simulink model "limited_time_undereacted_spacecraft_change"  (R2022a)
settings: Solver=ode4  StartTime=0.0  StopTime=30  FixedStep=0.001  RelTol=1e-11
libraries: simulink x4
settings Model: Creator=田佳怡  LastModifiedBy=lyuwenhao
settings SolverCC: AlgebraicLoopSolver=TrustRegion
settings DebuggingCC: UnconnectedInputMsg=warning  UnconnectedOutputMsg=warning  UnconnectedLineMsg=warning  SFMachineParentedDataDiag=warning
settings RTWCC: DLArmComputeVersion=19.05

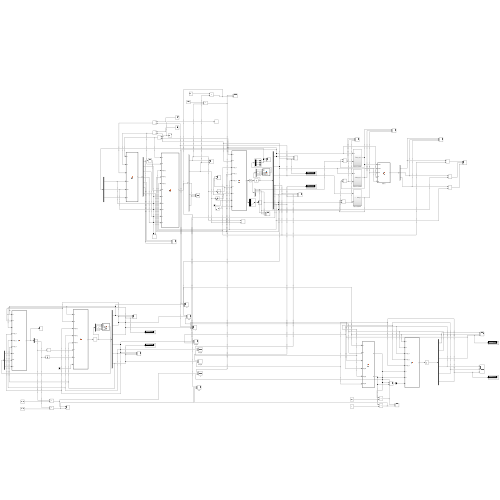
[thumbnail: Simulink's stored preview of the top-level diagram]
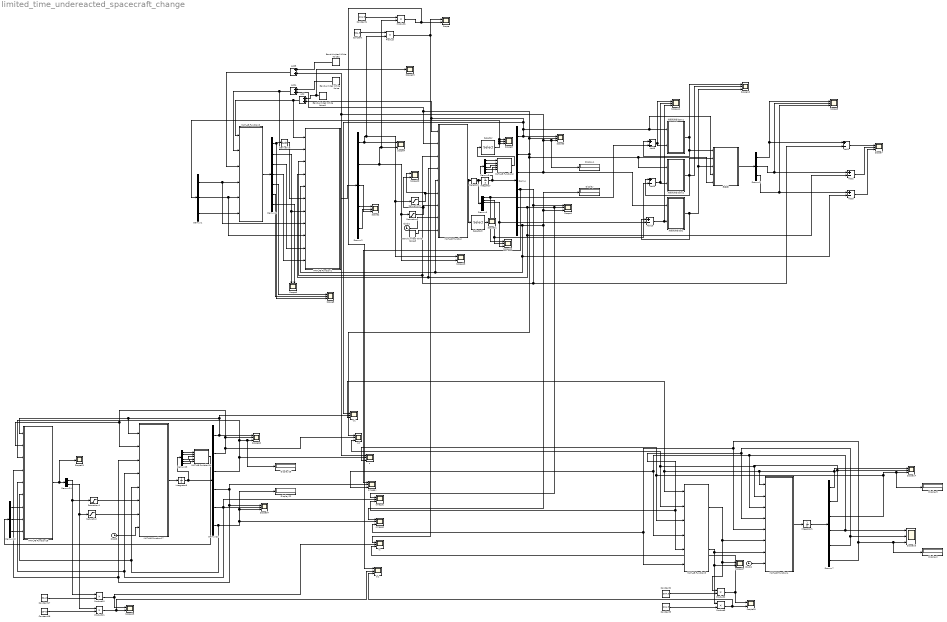
== system limited_time_undereacted_spacecraft_change ==
  Add : Sum
  Add{1..3,8..10} (6 alike) : Sum  Inputs=+-
  Add4 : Sum
  Add5 : Sum
  Band-Limited White Noise : simulink/Sources/Band-Limited White Noise  Cov=[0.001*0.001*0.0001]  Ts=0.01  seed=[23341]
  Band-Limited White Noise1 : simulink/Sources/Band-Limited White Noise  Cov=[0.001*0.001*0.0001]  Ts=0.01  seed=[23341]
  Band-Limited White Noise2 : simulink/Sources/Band-Limited White Noise  Cov=[0.001*0.001*0.0001]  Ts=0.1  seed=[23341]
  Band-Limited White Noise3 : simulink/Sources/Band-Limited White Noise  Cov=[0.001*0.001*0.0001]  Ts=0.01  seed=[23341]
  Clock1 : Clock
  Clock2 : Clock
  Clock3 : Clock
  Constant : Constant  Value=304.5
  Constant1 : Constant  Value=204.5
  Constant17 : Constant  Value=304.5
  Constant18 : Constant  Value=204.5
  Constant2 : Constant  Value=304.5
  Constant3 : Constant  Value=204.5
  Demux{,3,6..7,21,23} (6 alike) : Demux  Outputs=6
  Demux1 : Demux  Outputs=3
  Demux2 : Demux  Outputs=5
  Demux22 : Demux  Outputs=3
  Demux24 : Demux  Outputs=2
  Demux4 : Demux  Outputs=7
  Demux5 : Demux  Outputs=3
  Derivative : Derivative
  Display{,1..2,5,22,25} (6 alike) : Display
  Integrator : Integrator  InitialCondition=[2.5;2.5;-0.213175;0.1;-0.1;-0.15095622]
  Integrator1 : Integrator  InitialCondition=[2;2;0.428875;0.2;-0.2;-0.12250622]
  Integrator9 : Integrator  InitialCondition=[2;2;0.428875;0.2;-0.2;-0.12250622]
  MATLAB Function : MATLAB Function  TreatAsAtomicUnit=on
  MATLAB Function1 : MATLAB Function  TreatAsAtomicUnit=on
  MATLAB Function17 : MATLAB Function  TreatAsAtomicUnit=on
  MATLAB Function18 : MATLAB Function  TreatAsAtomicUnit=on
  MATLAB Function19 : MATLAB Function  TreatAsAtomicUnit=on
  MATLAB Function2 : MATLAB Function  TreatAsAtomicUnit=on
  MATLAB Function3 : MATLAB Function  TreatAsAtomicUnit=on
  MATLAB Function4 : MATLAB Function  TreatAsAtomicUnit=on
  MATLAB Function5 : MATLAB Function  TreatAsAtomicUnit=on
  Product{,1..3,10..11} (6 alike) : Product
  Saturation{,1..3} (4 alike) : Saturate
  Scope{,4,6,13,15,17..18,20} (8 alike) : Scope  NumInputPorts=2
  Scope{1..3,5,7..12,14,16,57,60} (14 alike) : Scope  NumInputPorts=3
  Scope19 : Scope
  Scope21 : Scope
  Scope61 : Scope
  Selector : Selector  InputPortWidth=3  IndexOptions=Index vector (dialog)  Indices=[1 2 3]  OutputSizes=1
  Selector1 : Selector  InputPortWidth=7  IndexOptions=Index vector (dialog)  Indices=[1 2 3 4 5 6]  OutputSizes=1
  Selector2 : Selector  InputPortWidth=7  IndexOptions=Index vector (dialog)  Indices=[7]  OutputSizes=1
  omegax : Scope  NumInputPorts=3
  omegay : Scope  NumInputPorts=3
  omegaz : Scope  NumInputPorts=3
  tx : Scope  NumInputPorts=3
  tx1 : Scope  NumInputPorts=3
  w1 : Scope  NumInputPorts=3
  w2 : Scope  NumInputPorts=3
  z : Scope  NumInputPorts=3
  滑膜观测器dotw1 : Subsystem
  滑膜观测器dotw2 : Subsystem
  滑膜观测器dotz : Subsystem
  角速度 : MATLAB Function  TreatAsAtomicUnit=on
  wires:
  Demux/3 -> z/1, Add5/2, Display1/1, Scope3/3, 滑膜观测器dotz/1(z)
  Demux/2 -> w2/1, 滑膜观测器dotw2/1(w2), 角速度/5(w2), Scope3/2, MATLAB Function/2(w2), Add4/2
  MATLAB Function1/1(y) -> Demux2/1
  MATLAB Function2/1(y) -> Selector/1
  Demux3/1 -> MATLAB Function2/1(w1)
  Demux3/2 -> MATLAB Function2/2(w2)
  Demux3/4 -> MATLAB Function2/3(omega_x)
  Demux3/5 -> MATLAB Function2/4(omega_y)
  Demux3/6 -> MATLAB Function2/5(omega_z)
  MATLAB Function3/1(y) -> Demux4/1
  Demux1/2 -> MATLAB Function1/9(dw2), MATLAB Function3/5(dw2)
  Demux1/1 -> MATLAB Function1/8(dw1), MATLAB Function3/4(dw1)
  Demux1/3 -> MATLAB Function3/6(dz)
  Demux4/1 -> Derivative/1, Scope5/3
  Derivative/1 -> MATLAB Function1/6(dz3)
  Demux4/2 -> MATLAB Function1/7(s2), Scope6/1
  Demux/4 -> Add1/2, MATLAB Function/3(omega_x), MATLAB Function1/3(omega_x), Scope1/1, omegax/1
  Demux4/3 -> MATLAB Function1/10(h1)
  Demux4/4 -> MATLAB Function1/11(h2)
  Constant/1 -> Product/1
  Product/1 -> Scope/1, tx/1
  Constant1/1 -> Product1/1
  Demux2/5 -> Scope2/2
  Demux2/4 -> Scope2/1
  Demux2/3 -> Scope2/3
  Demux4/5 -> Scope5/1
  Demux4/6 -> Scope5/2
  Selector/1 -> Scope8/3, Scope8/2, Scope8/1, Demux1/1
  Integrator/1 -> Demux/1, Demux3/1
  Demux5/3 -> Scope9/3, Add3/1
  角速度/1(y) -> Demux5/1
  Demux5/2 -> Scope9/2, Add2/1
  Demux5/1 -> Scope9/1, Add1/1
  Add8/1 -> Scope11/1, 滑膜观测器dotw1/2(In1)
  MATLAB Function/1(y) -> Selector2/1, Selector1/1
  Demux6/1 -> Scope12/1, Add8/2
  滑膜观测器dotw1/1(dotw_1估计) -> Scope10/1, 角速度/1(dotw1), Add8/1
  Add9/1 -> Scope11/2, 滑膜观测器dotw2/2(In1)
  Demux6/2 -> Scope12/2, Add9/2
  Add10/1 -> Scope11/3, 滑膜观测器dotz/2(In1)
  滑膜观测器dotz/1(dotz估计) -> Scope10/3, 角速度/3(dotz), Add10/1
  Demux6/3 -> Scope12/3, Add10/2
  滑膜观测器dotw2/1(dotw_2估计) -> 角速度/2(dotw2), Scope10/2, Add9/1
  Demux/6 -> Add3/2, MATLAB Function/5(omega_z), MATLAB Function1/5(omega_z), Display/1, Scope1/3, omegaz/1
  Add1/1 -> Scope7/1
  Add2/1 -> Scope7/2
  Add3/1 -> Scope7/3
  Demux4/7 -> Scope6/2
  Product11/1 -> tx1/2, Scope15/2
  Demux23/1 -> MATLAB Function19/1(w1)
  Demux22/3 -> MATLAB Function18/9(dz)
  Integrator9/1 -> Demux23/1, Demux21/1
  Demux22/1 -> MATLAB Function18/7(dw1)
  Demux21/4 -> MATLAB Function18/4(omega_x), MATLAB Function17/3(omega_x), Scope57/1, omegax/2
  Demux21/3 -> z/2, MATLAB Function18/3(z), Display25/1, Scope60/3
  MATLAB Function18/1(y) -> Scope61/1, Demux24/1
  Demux23/2 -> MATLAB Function19/2(w2)
  Constant17/1 -> Product10/2
  MATLAB Function17/1(y) -> Integrator9/1
  Demux22/2 -> MATLAB Function18/8(dw2)
  Demux23/4 -> MATLAB Function19/3(omega_x)
  MATLAB Function19/1(y) -> Demux22/1
  Demux24/1 -> Product10/1, Saturation1/1
  Demux24/2 -> Product11/1, Saturation/1
  Demux21/6 -> MATLAB Function17/5(omega_z), MATLAB Function18/6(omega_z), Display22/1, Scope57/3, omegaz/2
  Demux21/1 -> Scope60/1, w1/2, MATLAB Function18/1(w1), MATLAB Function17/1(w1)  "w1"
  Demux21/2 -> w2/2, Scope60/2, MATLAB Function18/2(w2), MATLAB Function17/2(w2)  "w2"
  Demux21/5 -> MATLAB Function17/4(omega_y), MATLAB Function18/5(omega_y), omegay/2, Scope57/2
  Constant18/1 -> Product11/2
  Demux23/6 -> MATLAB Function19/5(omega_z)
  Demux23/5 -> MATLAB Function19/4(omega_y)
  Demux7/2 -> MATLAB Function5/2(w2), w2/3, MATLAB Function4/2(w2), Scope14/2
  Demux7/1 -> MATLAB Function5/1(w1), w1/3, MATLAB Function4/1(w1), Scope14/1
  Demux7/3 -> MATLAB Function5/3(z), z/3, Display5/1, Scope14/3
  Clock2/1 -> MATLAB Function4/8(t)
  Demux7/6 -> MATLAB Function4/5(omega_z), MATLAB Function5/6(omegaz), omegaz/3, Display2/1, Scope16/3
  Integrator1/1 -> Demux7/1
  MATLAB Function4/1(y) -> Integrator1/1
  Demux/1 -> w1/1, MATLAB Function/1(w1), Add/2, 角速度/4(w1), 滑膜观测器dotw1/1(w1), Scope3/1
  Demux7/4 -> MATLAB Function4/3(omega_x), MATLAB Function5/4(omegax), omegax/3, Scope16/1
  Demux/5 -> Add2/2, MATLAB Function/4(omega_y), MATLAB Function1/4(omega_y), omegay/1, Scope1/2
  Demux7/5 -> MATLAB Function5/5(omegay), omegay/3, MATLAB Function4/4(omega_y), Scope16/2
  Product10/1 -> Scope15/1, tx/2
  Product2/1 -> Scope18/1, tx/3
  Constant3/1 -> Product3/2
  MATLAB Function5/2(u2) -> MATLAB Function4/7(u2), Product3/1, Scope17/2
  Constant2/1 -> Product2/2
  MATLAB Function5/1(u1) -> MATLAB Function4/6(u1), Product2/1, Scope17/1
  Product3/1 -> tx1/3, Scope18/2
  Product1/1 -> tx1/1, Scope/2
  Demux2/1 -> Scope13/1, Saturation3/1, Product/2, Scope4/1
  Demux2/2 -> Scope13/2, Saturation2/1, Scope4/2, Product1/2
  Clock1/1 -> MATLAB Function/8(t)
  Clock3/1 -> MATLAB Function17/8(t)
  Saturation1/1 -> MATLAB Function17/6(u1)
  Saturation/1 -> MATLAB Function17/7(u2)
  Band-Limited White Noise/1 -> Add4/1
  Band-Limited White Noise1/1 -> Scope19/1, Add/1
  Add/1 -> MATLAB Function3/1(w1), MATLAB Function1/1(w1)
  Add4/1 -> MATLAB Function3/2(w2), MATLAB Function1/2(w2)
  Band-Limited White Noise2/1 -> Add5/1
  Add5/1 -> MATLAB Function3/3(z)
  Saturation2/1 -> Scope20/2, MATLAB Function/7(u2)
  Saturation3/1 -> MATLAB Function/6(u1), Scope20/1
  Selector1/1 -> Demux6/1, Integrator/1
  Selector2/1 -> Scope21/1
  Band-Limited White Noise3/1 -> MATLAB Function/9(d)

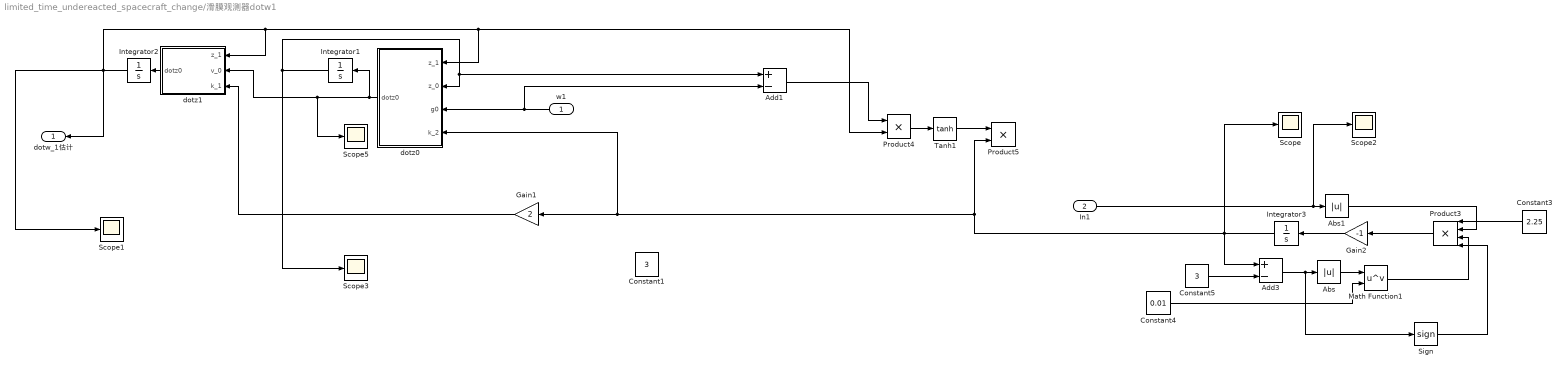
== system limited_time_undereacted_spacecraft_change/滑膜观测器dotw1 ==
  w1 : Inport
  In1 : Inport  Port=2
  Abs : Abs  SaturateOnIntegerOverflow=off
  Abs1 : Abs  SaturateOnIntegerOverflow=off
  Add1 : Sum  Inputs=+-
  Add3 : Sum  Inputs=+-
  Constant1 : Constant  Value=3
  Constant3 : Constant  Value=2.25
  Constant4 : Constant  Value=0.01
  Constant5 : Constant  Value=3
  Gain1 : Gain  Gain=2
  Gain2 : Gain  Gain=-1
  Integrator1 : Integrator
  Integrator2 : Integrator
  Integrator3 : Integrator  InitialCondition=8
  Math Function1 : Math  Operator=pow
  Product3 : Product  Inputs=4
  Product4 : Product
  Product5 : Product
  Scope{,1..3,5} (5 alike) : Scope
  Sign : Signum
  Tanh1 : Trigonometry  Operator=tanh
  dotz0 : MATLAB Function  TreatAsAtomicUnit=on
  dotz1 : MATLAB Function  TreatAsAtomicUnit=on
  dotw_1估计 : Outport
  wires:
  Tanh1/1 -> Product5/1
  Constant5/1 -> Add3/2
  Constant4/1 -> Math Function1/2
  w1/1 -> Add1/2, dotz0/3(g0)
  Product3/1 -> Gain2/1
  Constant3/1 -> Product3/1
  Gain2/1 -> Integrator3/1
  Add3/1 -> Sign/1, Abs/1
  Add1/1 -> Product4/1
  Integrator1/1 -> Scope3/1, dotz0/2(z_0), Add1/1
  Gain1/1 -> dotz1/3(k_1)
  Integrator2/1 -> dotw_1估计/1, Scope1/1, dotz0/1(z_1), Product4/2, dotz1/1(z_1)
  dotz1/1(dotz0) -> Integrator2/1
  In1/1 -> Scope2/1, Abs1/1
  Product4/1 -> Tanh1/1
  dotz0/1(dotz0) -> dotz1/2(v_0), Scope5/1, Integrator1/1
  Abs1/1 -> Product3/2
  Math Function1/1 -> Product3/3
  Abs/1 -> Math Function1/1
  Sign/1 -> Product3/4
  Integrator3/1 -> Scope/1, dotz0/4(k_2), Gain1/1, Product5/2, Add3/1

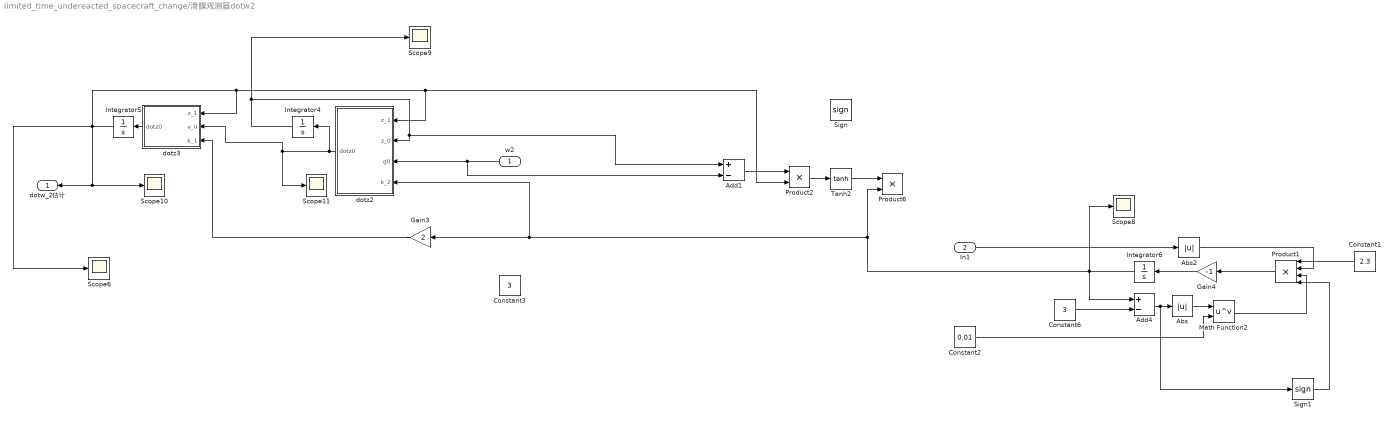
== system limited_time_undereacted_spacecraft_change/滑膜观测器dotw2 ==
  w2 : Inport
  In1 : Inport  Port=2
  Abs : Abs  SaturateOnIntegerOverflow=off
  Abs2 : Abs  SaturateOnIntegerOverflow=off
  Add1 : Sum  Inputs=+-
  Add4 : Sum  Inputs=+-
  Constant1 : Constant  Value=2.3
  Constant2 : Constant  Value=0.01
  Constant3 : Constant  Value=3
  Constant6 : Constant  Value=3
  Gain3 : Gain  Gain=2
  Gain4 : Gain  Gain=-1
  Integrator4 : Integrator
  Integrator5 : Integrator
  Integrator6 : Integrator  InitialCondition=8
  Math Function2 : Math  Operator=pow
  Product1 : Product  Inputs=4
  Product2 : Product
  Product6 : Product
  Scope{6,8..11} (5 alike) : Scope
  Sign : Signum
  Sign1 : Signum
  Tanh2 : Trigonometry  Operator=tanh
  dotz2 : MATLAB Function  TreatAsAtomicUnit=on
  dotz3 : MATLAB Function  TreatAsAtomicUnit=on
  dotw_2估计 : Outport
  wires:
  Tanh2/1 -> Product6/1
  Constant6/1 -> Add4/2
  Constant2/1 -> Math Function2/2
  w2/1 -> Add1/2, dotz2/3(g0)
  Product1/1 -> Gain4/1
  Constant1/1 -> Product1/1
  Gain4/1 -> Integrator6/1
  Add4/1 -> Sign1/1, Abs/1
  Add1/1 -> Product2/1
  Integrator4/1 -> Scope9/1, Add1/1, dotz2/2(z_0)
  Gain3/1 -> dotz3/3(k_1)
  Integrator5/1 -> dotw_2估计/1, Scope10/1, Scope6/1, dotz2/1(z_1), Product2/2, dotz3/1(z_1)
  dotz3/1(dotz0) -> Integrator5/1
  In1/1 -> Abs2/1
  Math Function2/1 -> Product1/3
  Product2/1 -> Tanh2/1
  Integrator6/1 -> dotz2/4(k_2), Gain3/1, Product6/2, Add4/1, Scope8/1
  dotz2/1(dotz0) -> dotz3/2(v_0), Scope11/1, Integrator4/1
  Abs2/1 -> Product1/2
  Abs/1 -> Math Function2/1
  Sign1/1 -> Product1/4

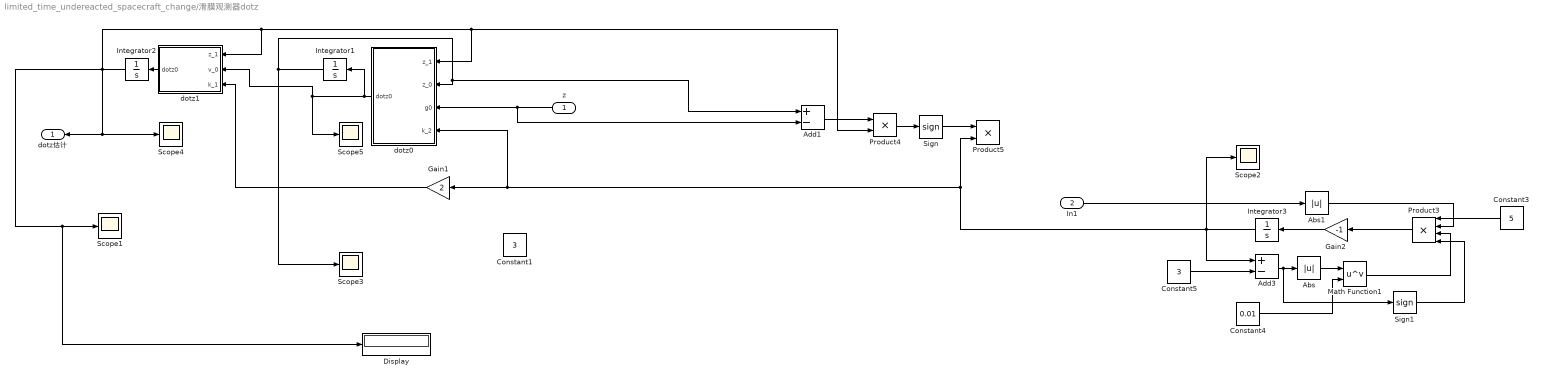
== system limited_time_undereacted_spacecraft_change/滑膜观测器dotz ==
  z : Inport
  In1 : Inport  Port=2
  Abs : Abs  SaturateOnIntegerOverflow=off
  Abs1 : Abs  SaturateOnIntegerOverflow=off
  Add1 : Sum  Inputs=+-
  Add3 : Sum  Inputs=+-
  Constant1 : Constant  Value=3
  Constant3 : Constant  Value=5
  Constant4 : Constant  Value=0.01
  Constant5 : Constant  Value=3
  Display : Display
  Gain1 : Gain  Gain=2
  Gain2 : Gain  Gain=-1
  Integrator1 : Integrator
  Integrator2 : Integrator
  Integrator3 : Integrator  InitialCondition=8
  Math Function1 : Math  Operator=pow
  Product3 : Product  Inputs=4
  Product4 : Product
  Product5 : Product
  Scope{1..5} (5 alike) : Scope
  Sign : Signum
  Sign1 : Signum
  dotz0 : MATLAB Function  TreatAsAtomicUnit=on
  dotz1 : MATLAB Function  TreatAsAtomicUnit=on
  dotz估计 : Outport
  wires:
  dotz0/1(dotz0) -> dotz1/2(v_0), Scope5/1, Integrator1/1
  dotz1/1(dotz0) -> Integrator2/1
  Gain1/1 -> dotz1/3(k_1)
  Product4/1 -> Sign/1
  Integrator1/1 -> Scope3/1, Add1/1, dotz0/2(z_0)
  z/1 -> Add1/2, dotz0/3(g0)
  Sign/1 -> Product5/1
  Add1/1 -> Product4/1
  Integrator2/1 -> dotz估计/1, Scope4/1, Display/1, Scope1/1, dotz0/1(z_1), Product4/2, dotz1/1(z_1)
  Integrator3/1 -> dotz0/4(k_2), Gain1/1, Product5/2, Add3/1, Scope2/1
  Constant4/1 -> Math Function1/2
  Math Function1/1 -> Product3/3
  Add3/1 -> Sign1/1, Abs/1
  In1/1 -> Abs1/1
  Abs1/1 -> Product3/2
  Constant5/1 -> Add3/2
  Gain2/1 -> Integrator3/1
  Constant3/1 -> Product3/1
  Product3/1 -> Gain2/1
  Abs/1 -> Math Function1/1
  Sign1/1 -> Product3/4

== matlab function limited_time_undereacted_spacecraft_change/MATLAB Function5 ==
  data: w1 input; u1 output; w2 input; z input; omegax input; omegay input; omegaz input; u2 output
function [u1, u2] = fcn(w1, w2, z, omegax, omegay, omegaz)

J3 = 403.6; J1= 304.5; J2 = 204.5; a1 = (J2 - J3) / J1; a2 = (J3 - J1) / J2; a3 = (J1 - J2) / J3;
k1 = 0.5; k2 = 0.5; k3 = 2; m = 10; n = 5; ks = 0.8; epsilon = 0.01;

v1 = omegax+k1*w1;
v2 = omegay+k2*w2;

u_eq1 = -k1*(w2*omegaz + 0.5*(1+w1^2-w2^2)*omegax + w1*w2*omegay) - ks*v1-epsilon*tanh(v1) - a1*omegay*omegaz;

u_eq2 = -k2*(-w1*omegaz + 0.5*(1-w1^2+w2^2)*omegay + w1*w2*omegax) - ks*v2-epsilon*tanh(v2) - a2*omegax*omegaz;

% us = (-ks*s2-epsilon*sign(s2)-h2*v3_dot) / (R_omegax+h1*R_omegay);

u1 = u_eq1;
u2 = u_eq2;

end

== matlab function limited_time_undereacted_spacecraft_change/滑膜观测器dotw1/dotz0 ==
  data: z_1 input; z_0 input; dotz0 output; g0 input; k_2 input
function dotz0 = fcn(z_1, z_0, g0, k_2)

v_0 = z_1 - k_2*abs(z_0 - g0)^(0.5)*tanh(z_0 - g0);


dotz0 = v_0;

== matlab function limited_time_undereacted_spacecraft_change/滑膜观测器dotw1/dotz1 ==
  data: z_1 input; dotz0 output; v_0 input; k_1 input
function dotz0 = fcn(z_1, v_0, k_1)


u = -k_1*tanh(z_1 - v_0);


dotz0 = u;

== matlab function limited_time_undereacted_spacecraft_change/滑膜观测器dotw2/dotz2 ==
  data: z_1 input; z_0 input; dotz0 output; g0 input; k_2 input
function dotz0 = fcn(z_1, z_0, g0, k_2)

v_0 = z_1 - k_2*abs(z_0 - g0)^(0.5)*tanh(z_0 - g0);


dotz0 = v_0;

== matlab function limited_time_undereacted_spacecraft_change/滑膜观测器dotw2/dotz3 ==
  data: z_1 input; dotz0 output; v_0 input; k_1 input
function dotz0 = fcn(z_1, v_0, k_1)


u = -k_1*tanh(z_1 - v_0);


dotz0 = u;

== matlab function limited_time_undereacted_spacecraft_change/滑膜观测器dotz/dotz0 ==
  data: z_1 input; z_0 input; dotz0 output; g0 input; k_2 input
function dotz0 = fcn(z_1, z_0, g0, k_2)

v_0 = z_1 - k_2*abs(z_0 - g0)^(0.5)*tanh(z_0 - g0);


dotz0 = v_0;

== matlab function limited_time_undereacted_spacecraft_change/滑膜观测器dotz/dotz1 ==
  data: z_1 input; dotz0 output; v_0 input; k_1 input
function dotz0 = fcn(z_1, v_0, k_1)


u = -k_1*tanh(z_1 - v_0);


dotz0 = u;

== matlab function limited_time_undereacted_spacecraft_change/角速度 ==
  data: dotw1 input; y output; dotw2 input; dotz input; w1 input; w2 input
function y = fcn(dotw1, dotw2, dotz, w1, w2)

% if(data<0.155)
    omega1 = (2*dotw1 - 2*dotz*w2 ) / (1+w1^2+w2^2);

    omega2 = (2*dotw2 + 2*dotz*w1 ) / (1+w1^2+w2^2);

    omega3 = dotz-w1*omega2+w2*omega1;
% else
%      omega1 = (2*dotw1-w2*(2*dotz-4*w1*dotw2)+4*w1^2*dotw1)/(1+w1^2+w2^2) - (4*w1*(w1*dotw1+w2*dotw2))/(w1^2+w2^2);
% 
%      omega2 = (2*dotw2-w1*(2*dotz+4*dotw1*w2)+4*w2^2*dotw2)/(1+w1^2+w2^2) - (4*w2*(w1*dotw1+w2*dotw2))/(w1^2+w2^2);
% 
%      omega3 = dotz-2*(dotz*w1^2+dotw2*w1+dotz*w2^2-dotw1*w2);
% end
    

y = [omega1; omega2; omega3];

== matlab function limited_time_undereacted_spacecraft_change/MATLAB Function17 ==
  data: w1 input; y output; w2 input; omega_x input; omega_y input; omega_z input; u1 input; u2 input; t input
function y = fcn(w1,w2,omega_x,omega_y,omega_z,u1,u2, t)

Jx = 304.5; Jy = 403.6; Jz = 204.5;

w1_dot = w2*omega_z + 0.5*(1+w1^2-w2^2)*omega_x + w1*w2*omega_y;
w2_dot = -w1*omega_z + 0.5*(1-w1^2+w2^2)*omega_y + w1*w2*omega_x;
z_dot = omega_z + w1*omega_y - w2*omega_x;

d1 = (1.6*sin(1.5*t)+0.3)/Jx;
d2 = (1.8*cos(1.2*t)+0.2)/Jy;

omega_x_dot = ((Jy-Jz)/Jx)*omega_y*omega_z + u1 + d1;
omega_y_dot = ((Jz-Jx)/Jy)*omega_x*omega_z + u2 + d2;
omega_z_dot = ((Jx-Jy)/Jz)*omega_x*omega_y; 

y = [w1_dot;w2_dot;z_dot;omega_x_dot;omega_y_dot;omega_z_dot];

== matlab function limited_time_undereacted_spacecraft_change/MATLAB Function18 ==
  data: w1 input; y output; w2 input; z input; omega_x input; omega_y input; omega_z input; dw1 input; dw2 input; dz input
function y = fcn(w1,w2,z,omega_x,omega_y,omega_z,dw1,dw2,dz)

Jx = 304.5; Jy = 204.5; Jz = 403.6;
k1 = 2; k2 = 2; h1 = 1; h2 = 1; alpha1 = 9/11;
alpha2 = 2*alpha1/(alpha1+1);
beta1 = 2*alpha1+1;
beta2 = (2*alpha1+1)/(alpha1+1);

kesai_x = -4*Jx*(w1*dw1^2-w1*w2*dw1*dz+w2*dw1*dw2-w2^2*dw2*dz)/(1+w1^2+w2^2)...
          + (Jz-Jy)*(1+w1^2+w2^2)*omega_y*omega_z;

kesai_y = -4*Jy*(w1*dw1*dw2+w1^2*dw1*dz+w2*dw2^2+w1^2*dw1*dz)/(1+w1^2+w2^2)...
          + (Jx-Jz)*(1+w1^2+w2^2)*omega_x*omega_z;

kesai_z = -4*Jz*(w1*dw1+w2*dw2)*(-w1*dw2+w2*dw1+dz/2*(1-w1^2-w2^2))/(1+w1^2+w2^2)...
          + (Jy-Jx)*(1+w1^2+w2^2)*omega_x*omega_y;

kesai1 = w2*(Jy*Jz*w2*kesai_x-Jx*Jz*w1*kesai_y-Jx*Jy*kesai_z)/((Jx*Jy*Jz)*(1+w1^2+w2^2))...
         +dw2*dz - kesai_x/(2*Jx);

kesai2 = w1*(Jy*Jz*w2*kesai_x-Jx*Jz*w1*kesai_y+Jx*Jy*kesai_z)/((Jx*Jy*Jz)*(1+w1^2+w2^2))...
         -dw1*dz - kesai_y/(2*Jy);

kesai3 = (Jy*Jz*w2*kesai_x-Jx*Jz*w1*kesai_y-Jx*Jy*kesai_z)/((Jx*Jy*Jz)*(1+w1^2+w2^2));

u1 = -k1*(abs(w1))^alpha1*sign(w1) - k2*(abs(dw1))^alpha2*sign(dw1) ...
     - h1*(abs(w1))^beta1*sign(w1) - h2*(abs(dw1))^beta2*sign(dw1) - kesai1;

u2 = -k1*(abs(w2))^alpha1*sign(w2) - k2*(abs(dw2))^alpha2*sign(dw2) ...
     - h1*(abs(w2))^beta1*sign(w2) - h2*(abs(dw2))^beta2*sign(dw2) - kesai2;

y = [u1;u2];

== matlab function limited_time_undereacted_spacecraft_change/MATLAB Function19 ==
  data: w1 input; y output; w2 input; omega_x input; omega_y input; omega_z input
function y = fcn(w1,w2,omega_x,omega_y,omega_z)

% if(w1^2+w2^2>1.0)
%     w1=w1/(w1^2+w2^2);
%     w2=w2/(w1^2+w2^2);
% end

w1_dot = w2*omega_z + 0.5*(1+w1^2-w2^2)*omega_x + w1*w2*omega_y;
w2_dot = -w1*omega_z + 0.5*(1-w1^2+w2^2)*omega_y + w1*w2*omega_x;
z_dot = omega_z + w1*omega_y - w2*omega_x;

% w1_dot = w2*omega_z - 0.5*(1+w1^2-w2^2)*omega_x - w1*w2*omega_y;
% w2_dot = -w1*omega_z - 0.5*(1-w1^2+w2^2)*omega_y - w1*w2*omega_x;
% z_dot = omega_z + (w1/(w1^2+w2^2))*omega_y - (w2/(w1^2+w2^2))*omega_x;

y = [w1_dot;w2_dot;z_dot];

== matlab function limited_time_undereacted_spacecraft_change/MATLAB Function1 ==
  data: w1 input; w2 input; omega_x input; omega_y input; omega_z input; dz3 input; y output; s2 input; dw1 input; dw2 input; h1 input; h2 input
function y = fcn(w1,w2,omega_x,omega_y,omega_z,dz3,s2,dw1,dw2,h1,h2)

Jx = 304.5; Jy = 204.5; Jz = 403.6;
k1 = 12; k2 = 12; p = 0.01; c=4;
ks = 10;epsilon = 0.001;

a1 = ((Jy-Jz)/Jx);
a2 = ((Jz-Jx)/Jy);
a3 = ((Jx-Jy)/Jz);

us = -(2*h2*dz3+2*ks*s2+2*epsilon*tanh(s2/c^2)) / ((w1^2-w2^2)*(1-h1)+(2*w1*w2+1)*(h1+1)); 

sigma1 = abs(w1)^(p - 1);
sigma2 = abs(w2)^(p - 1);
 
u1 = -a1*omega_y*omega_z + us + ...
     (2*w2*((omega_y+omega_z*w1+k1*p*sigma1*w2)*dw1+(-omega_x+omega_z*w2-k2*p*sigma2*w1)*dw2+a3*omega_x*omega_y)) / (w1^2+w2^2-18) - ...
     (2*dw1*(omega_x*w1+k1*p*sigma1+omega_z*w1*w2+k1*p*sigma1*w2^2)+2*dw2*(omega_z+omega_z*w2^2+omega_y*w1-k2*p*sigma2*w1*w2)) / (w1^2+w2^2+1);

u2 = -a2*omega_z*omega_x + us - ...
    (2*w1*((omega_y+omega_z*w1+k1*p*sigma1*w2)*dw1+(-omega_x+omega_z*w2-k2*p*sigma2*w1)*dw2+a3*omega_x*omega_y)) / (w1^2+w2^2-18) + ...
    (2*dw2*(-omega_y*w2-k2*p*sigma2+omega_z*w1*w2-k2*p*sigma2*w1^2)+2*dw1*(omega_z+omega_z*w1^2-omega_x*w2+k1*p*sigma1*w1*w2)) / (w1^2+w2^2+1);

u_eq1=u1-us;
u_eq2=u2-us;

y = [u1;u2;us;u_eq1;u_eq2];

== matlab function limited_time_undereacted_spacecraft_change/MATLAB Function ==
  data: w1 input; y output; w2 input; omega_x input; omega_y input; omega_z input; u1 input; u2 input; t input; d input
function y = fcn(w1,w2,omega_x,omega_y,omega_z,u1,u2, t, d)

Jx = 304.5; Jy = 204.5; Jz = 403.6;

w1_dot = w2*omega_z + 0.5*(1+w1^2-w2^2)*omega_x + w1*w2*omega_y;
w2_dot = -w1*omega_z + 0.5*(1-w1^2+w2^2)*omega_y + w1*w2*omega_x;
z_dot = omega_z + w1*omega_y - w2*omega_x;
d1 = (1.6*sin(1.5*t)+0.3)/Jx;
d2 = (1.8*cos(1.2*t)+0.2)/Jy;

omega_x_dot = ((Jy-Jz)/Jx)*omega_y*omega_z + u1 + d1+d;
omega_y_dot = ((Jz-Jx)/Jy)*omega_x*omega_z + u2 + d2+d;
omega_z_dot = ((Jx-Jy)/Jz)*omega_x*omega_y; 

y = [w1_dot;w2_dot;z_dot;omega_x_dot;omega_y_dot;omega_z_dot;d1];

== matlab function limited_time_undereacted_spacecraft_change/MATLAB Function2 ==
  data: w1 input; y output; w2 input; omega_x input; omega_y input; omega_z input
function y = fcn(w1,w2,omega_x,omega_y,omega_z)

% if(w1^2+w2^2>1.0)
%     w1=w1/(w1^2+w2^2);
%     w2=w2/(w1^2+w2^2);
% end

w1_dot = w2*omega_z + 0.5*(1+w1^2-w2^2)*omega_x + w1*w2*omega_y;
w2_dot = -w1*omega_z + 0.5*(1-w1^2+w2^2)*omega_y + w1*w2*omega_x;
z_dot = omega_z + w1*omega_y - w2*omega_x;

% w1_dot = w2*omega_z - 0.5*(1+w1^2-w2^2)*omega_x - w1*w2*omega_y;
% w2_dot = -w1*omega_z - 0.5*(1-w1^2+w2^2)*omega_y - w1*w2*omega_x;
% z_dot = omega_z + (w1/(w1^2+w2^2))*omega_y - (w2/(w1^2+w2^2))*omega_x;

y = [w1_dot;w2_dot;z_dot];

== matlab function limited_time_undereacted_spacecraft_change/MATLAB Function3 ==
  data: w1 input; y output; w2 input; z input; dw1 input; dw2 input; dz input
function y = fcn(w1,w2,z,dw1,dw2,dz)

k1 = 12; k2 = 12; k3 = 5; p = 0.01; c=4;
m = 10; n = 5;

z1 = dw1 + k1*(abs(w1))^p*tanh(w1/c^2);
z2 = dw2 + k2*(abs(w2))^p*tanh(w2/c^2);
z3 = dz + k3*(abs(z))^p*tanh(z/c^2);

h1 = m*tanh((z1*z2)/c^2);
s1 = z1 + h1*z2;
h2 = n*tanh((s1*z3)/c^2);
s2 = s1 + h2*z3;

y = [z3;s2;h1;h2;z1;z2;s1];

== matlab function limited_time_undereacted_spacecraft_change/MATLAB Function4 ==
  data: w1 input; y output; w2 input; omega_x input; omega_y input; omega_z input; u1 input; u2 input; t input
function y = fcn(w1,w2,omega_x,omega_y,omega_z,u1,u2, t)

Jx = 304.5; Jy = 204.5; Jz = 403.6;

w1_dot = w2*omega_z + 0.5*(1+w1^2-w2^2)*omega_x + w1*w2*omega_y;
w2_dot = -w1*omega_z + 0.5*(1-w1^2+w2^2)*omega_y + w1*w2*omega_x;
if (t<=30)
    z_dot = omega_z + w1*omega_y - w2*omega_x;
else
    z_dot = omega_z + w1/(w1^2+w2^2)*omega_y - w2/(w1^2+w2^2)*omega_x;
end

d1 = (1.6*sin(1.5*t)+0.3)/Jx;
d2 = (1.8*cos(1.2*t)+0.2)/Jy;

omega_x_dot = ((Jy-Jz)/Jx)*omega_y*omega_z + u1 + d1*1;
omega_y_dot = ((Jz-Jx)/Jy)*omega_x*omega_z + u2 + d2*1;
omega_z_dot = ((Jx-Jy)/Jz)*omega_x*omega_y; 

y = [w1_dot;w2_dot;z_dot;omega_x_dot;omega_y_dot;omega_z_dot];
